simulink model "model"  (R2023a)
settings: Solver=VariableStepAuto  StartTime=0.0  StopTime=10  RelTol=1e-3
values from neighbouring files (symbols this model uses):
  Am = A - b*k    [main.m]
  Bm = b    [main.m]
  ga = diag([100,100,100,100])    [main.m]
  gb = 100    [main.m]
  J1 = 0.005    [main.m]
  J2 = 0.1    [main.m]
  k = acker(A,b,P)    [main.m]
  ke = 1    [main.m]
  km = 1    [main.m]
  kn = 1/(-C/(A-b*k)*b)    [main.m]
  L = 0.01    [main.m]
  P = P3    [main.m]
  p = 0.5    [main.m]
  R = 2    [main.m]
settings Model: Creator=User  LastModifiedBy=User

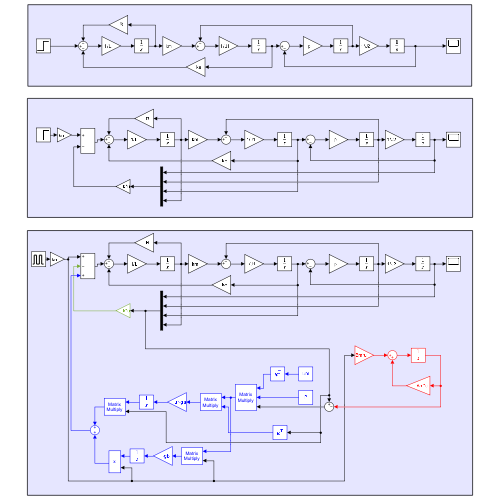
[thumbnail: Simulink's stored preview of the top-level diagram]
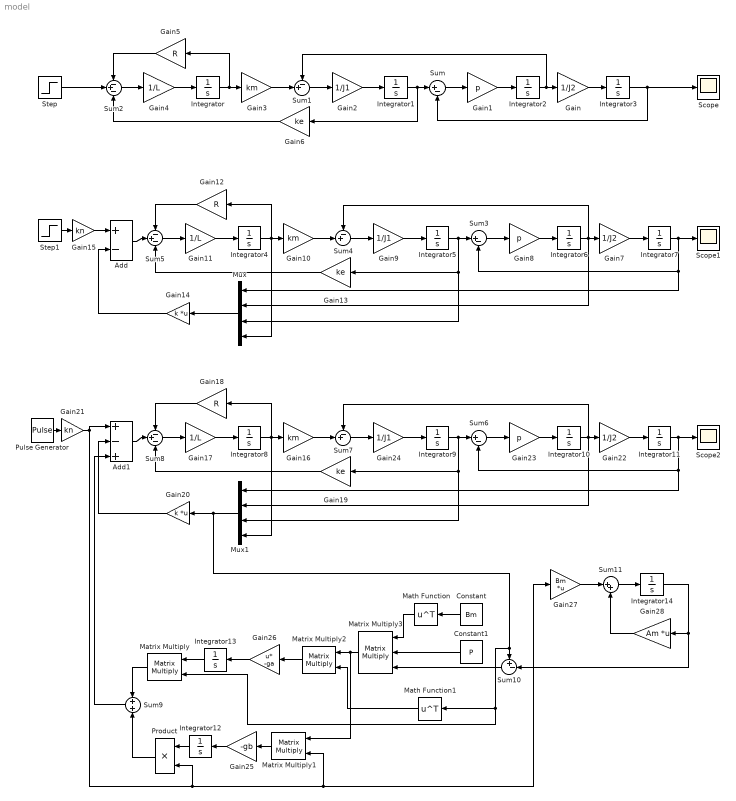
== system model ==
  Add : Sum  Inputs=+-
  Add1 : Sum  Inputs=+-+
  Constant : Constant  Value=Bm  VectorParams1D=off
  Constant1 : Constant  Value=P  VectorParams1D=off
  Gain : Gain  Gain=1/J2
  Gain1 : Gain  Gain=p
  Gain10 : Gain  Gain=km
  Gain11 : Gain  Gain=1/L
  Gain12 : Gain  Gain=R
  Gain13 : Gain  Gain=ke
  Gain14 : Gain  Gain=k  Multiplication=Matrix(K*u)
  Gain15 : Gain  Gain=kn
  Gain16 : Gain  Gain=km
  Gain17 : Gain  Gain=1/L
  Gain18 : Gain  Gain=R
  Gain19 : Gain  Gain=ke
  Gain2 : Gain  Gain=1/J1
  Gain20 : Gain  Gain=k  Multiplication=Matrix(K*u)
  Gain21 : Gain  Gain=kn
  Gain22 : Gain  Gain=1/J2
  Gain23 : Gain  Gain=p
  Gain24 : Gain  Gain=1/J1
  Gain25 : Gain  Gain=-gb
  Gain26 : Gain  Gain=-ga  Multiplication=Matrix(u*K)
  Gain27 : Gain  Gain=Bm  Multiplication=Matrix(K*u)
  Gain28 : Gain  Gain=Am  Multiplication=Matrix(K*u)
  Gain3 : Gain  Gain=km
  Gain4 : Gain  Gain=1/L
  Gain5 : Gain  Gain=R
  Gain6 : Gain  Gain=ke
  Gain7 : Gain  Gain=1/J2
  Gain8 : Gain  Gain=p
  Gain9 : Gain  Gain=1/J1
  Integrator{,1..14} (15 alike) : Integrator
  Math Function : Math  Operator=transpose
  Math Function1 : Math  Operator=transpose
  Matrix Multiply : Product  Multiplication=Matrix(*)
  Matrix Multiply1 : Product  Multiplication=Matrix(*)
  Matrix Multiply2 : Product  Multiplication=Matrix(*)
  Matrix Multiply3 : Product  Inputs=3  Multiplication=Matrix(*)
  Mux : Mux
  Mux1 : Mux
  Product : Product
  Pulse Generator : DiscretePulseGenerator  PulseType=Time based  Period=5  PulseWidth=50
  Scope : Scope
  Scope1 : Scope
  Scope2 : Scope
  Step : Step  Time=0  SampleTime=0
  Step1 : Step  Time=0  SampleTime=0
  Sum : Sum  Inputs=|+-
  Sum1 : Sum  Inputs=-+|
  Sum10 : Sum  Inputs=+-|
  Sum11 : Sum  Inputs=|++
  Sum2 : Sum  Inputs=-+-
  Sum3 : Sum  Inputs=|+-
  Sum4 : Sum  Inputs=-+|
  Sum5 : Sum  Inputs=-+-
  Sum6 : Sum  Inputs=|+-
  Sum7 : Sum  Inputs=-+|
  Sum8 : Sum  Inputs=-+-
  Sum9 : Sum
  wires:
  Gain1/1 -> Integrator2/1
  Step/1 -> Sum2/2
  Gain3/1 -> Sum1/2
  Integrator/1 -> Gain5/1, Gain3/1
  Gain5/1 -> Sum2/1
  Integrator3/1 -> Scope/1, Sum/2
  Integrator1/1 -> Gain6/1, Sum/1
  Sum/1 -> Gain1/1
  Sum1/1 -> Gain2/1
  Gain6/1 -> Sum2/3
  Gain4/1 -> Integrator/1
  Integrator2/1 -> Sum1/1, Gain/1
  Gain2/1 -> Integrator1/1
  Gain/1 -> Integrator3/1
  Sum2/1 -> Gain4/1
  Gain9/1 -> Integrator5/1
  Integrator6/1 -> Mux/2, Sum4/1, Gain7/1
  Gain13/1 -> Sum5/3
  Sum3/1 -> Gain8/1
  Integrator5/1 -> Gain13/1, Mux/3, Sum3/1
  Integrator7/1 -> Scope1/1, Mux/1, Sum3/2
  Gain7/1 -> Integrator7/1
  Gain11/1 -> Integrator4/1
  Sum4/1 -> Gain9/1
  Gain10/1 -> Sum4/2
  Gain8/1 -> Integrator6/1
  Integrator4/1 -> Mux/4, Gain12/1, Gain10/1
  Gain12/1 -> Sum5/1
  Sum5/1 -> Gain11/1
  Add/1 -> Sum5/2
  Mux/1 -> Gain14/1
  Gain14/1 -> Add/2
  Step1/1 -> Gain15/1
  Gain15/1 -> Add/1
  Add1/1 -> Sum8/2
  Sum8/1 -> Gain17/1
  Gain17/1 -> Integrator8/1
  Gain23/1 -> Integrator10/1
  Sum7/1 -> Gain24/1
  Gain18/1 -> Sum8/1
  Integrator8/1 -> Mux1/4, Gain18/1, Gain16/1
  Gain22/1 -> Integrator11/1
  Integrator9/1 -> Gain19/1, Mux1/3, Sum6/1
  Gain21/1 -> Matrix Multiply1/2, Gain27/1, Product/2, Add1/1
  Gain20/1 -> Add1/2
  Gain16/1 -> Sum7/2
  Gain19/1 -> Sum8/3
  Sum6/1 -> Gain23/1
  Integrator10/1 -> Mux1/2, Sum7/1, Gain22/1
  Mux1/1 -> Sum10/1, Math Function1/1, Matrix Multiply/2, Gain20/1
  Gain24/1 -> Integrator9/1
  Integrator11/1 -> Scope2/1, Mux1/1, Sum6/2
  Matrix Multiply/1 -> Sum9/1
  Product/1 -> Sum9/2
  Integrator12/1 -> Product/1
  Gain25/1 -> Integrator12/1
  Matrix Multiply1/1 -> Gain25/1
  Sum9/1 -> Add1/3
  Integrator13/1 -> Matrix Multiply/1
  Gain26/1 -> Integrator13/1
  Matrix Multiply2/1 -> Gain26/1
  Matrix Multiply3/1 -> Matrix Multiply1/1, Matrix Multiply2/1
  Math Function/1 -> Matrix Multiply3/1
  Constant/1 -> Math Function/1
  Constant1/1 -> Matrix Multiply3/2
  Sum10/1 -> Matrix Multiply3/3
  Math Function1/1 -> Matrix Multiply2/2
  Gain27/1 -> Sum11/1
  Sum11/1 -> Integrator14/1
  Gain28/1 -> Sum11/2
  Integrator14/1 -> Sum10/2, Gain28/1
  Pulse Generator/1 -> Gain21/1
